simulink model "nonlinear_sys"  (R2017a)
settings: Solver=VariableStepAuto  StartTime=0.0  StopTime=10  RelTol=1e-3
undefined symbols (not defined in the file or in its folder): DC, NC
settings Model: Creator=julio  LastModifiedBy=julio

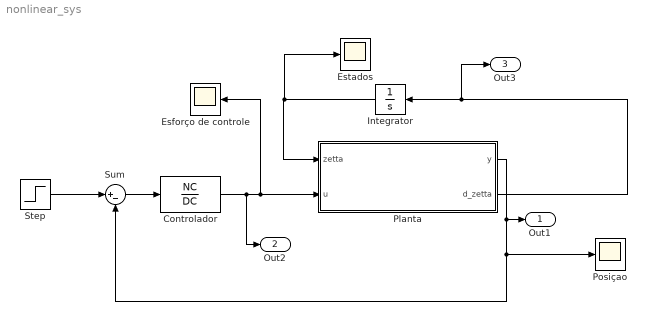
== system nonlinear_sys ==
  Controlador : TransferFcn  Numerator=NC  Denominator=DC  ContinuousStateAttributes='Controler'
  Esforço de controle : Scope
  Estados : Scope
  Integrator : Integrator  InitialCondition=[0 0 0 0]
  Planta : MATLAB Function  RequirementInfo="{}  %GIDa_0630ebdc_7833_47fa_aec0_145c00fbcbb1"  TreatAsAtomicUnit=on  RTWFcnName=nonlinear_func  RTWFileName=nonlinear_func
      settings: RTWFileNameOpts=User specified
  Posiçao : Scope
  Step : Step  Time=0  After=10  SampleTime=0
  Sum : Sum  Inputs=|+-
  Out1 : Outport  SignalName=y
  Out2 : Outport  Port=2  SignalName=esf
  Out3 : Outport  Port=3  SignalName=state
  wires:
  Controlador/1 -> Out2/1, Esforço de controle/1, Planta/2(u)
  Step/1 -> Sum/1
  Sum/1 -> Controlador/1
  Planta/2(d_zetta) -> Out3/1, Integrator/1
  Integrator/1 -> Estados/1, Planta/1(zetta)
  Planta/1(y) -> Out1/1, Sum/2, Posiçao/1

== matlab function nonlinear_sys/Planta ==
  data: zetta input size=4; u input size=1; y output size=1; d_zetta output size=4
function [ y, d_zetta] = nonlinear_func(zetta, u)
%UNTITLED Summary of this function goes here
%   Detailed explanation goes here
    
    MJ = 1.0731; % [kg]
    m  = 0.209;  % [kg]
    l  = 0.3302; % [m]
    bK = 5.4;    % [N.s/(m²)]
    Kr = 1.0717; % [N/V]
    g  = 9.81;   % [m/s^2]

    M_aux = MJ + m*sin(zetta(3))^2;
    
    A = [ 0 1 0 0
          0 -bK/M_aux 0 -(m*l*zetta(4)*sin(zetta(3)))/M_aux
          0 0 0 1
          0 bK*cos(zetta(3))/(M_aux*l) 0 -m*zetta(4)*sin(zetta(3))*cos(zetta(3))/(M_aux)];
      
    F1 = m*g*sin(zetta(3))*cos(zetta(3)) + Kr*u;
    F2 = -cos(zetta(3))*F1/(l*M_aux) - g*sin(zetta(3))/l;
    
    B = [ 0 F1/M_aux 0 F2]';
    
    y = zetta(1);
    d_zetta = A*zetta + B;

end
